simulink model "uz_ssi_interface"  (R2021a)
settings: Solver=FixedStepDiscrete  StartTime=0.0  StopTime=1200e-6  RelTol=1e-3
values from neighbouring files (symbols this model uses):
  f_ADC = 50e3    (= 50000)    [uz_ssi_interface_init.m]
  f_clock = 100e6    (= 100000000)    [uz_ssi_interface_init.m]
  ssi_encoder_bit_width = 17    [uz_ssi_interface_init.m]
  t_clock = 1/f_clock    (= 1e-08)    [uz_ssi_interface_init.m]
libraries: hdlsllib x21, simulink x10, simulink_extras x3, dspsigops x1
settings Model: DataTypeOverride=Off  Creator=micha  LastModifiedBy=micha
settings SolverCC: AlgebraicLoopSolver=TrustRegion
settings DataIOCC: LimitDataPoints=on  SaveOutput=off  SaveTime=off
settings OptimizationCC: BlockReduction=off  ConditionallyExecuteInputs=off  DefaultParameterBehavior=Inlined  LifeSpan=inf
settings DebuggingCC: AlgebraicLoopMsg=error  SingleTaskRateTransMsg=error  AllowSymbolicDim=off  StrictBusMsg=ErrorOnBusTreatedAsVector  SFUnexpectedBacktrackingDiag=warning  SFNoUnconditionalDefaultTransitionDiag=warning  SFExecutionAtInitializationDiag=none  SFMachineParentedDataDiag=warning  ArithmeticOperatorsInVariantConditions=warning
settings HardwareCC: ProdBitPerPointer=32  ProdBitPerSizeT=32  ProdBitPerPtrDiffT=32  ProdLargestAtomicFloat=None  ProdIntDivRoundTo=Undefined  ProdEndianess=Unspecified  ProdWordSize=32  ProdHWDeviceType=ASIC/FPGA->ASIC/FPGA  ProdEqTarget=off
settings SFSimCC: SimUseLocalCustomCode=off  CustomCodeUndefinedFunction=UseInterfaceOnly
settings RTWCC: RTWUseLocalCustomCode=off
settings CodeAppCC: StateflowObjectComments=on
settings GRTTargetCC: TargetLangStandard=C89/C90 (ANSI)
settings ConfigComp: CovScope=ReferencedModels  CovMetricSettings=dw  CovSaveCumulativeToWorkspaceVar=on  CovSaveSingleToWorkspaceVar=on  CovExternalEMLEnable=off  CovSFcnEnable=off

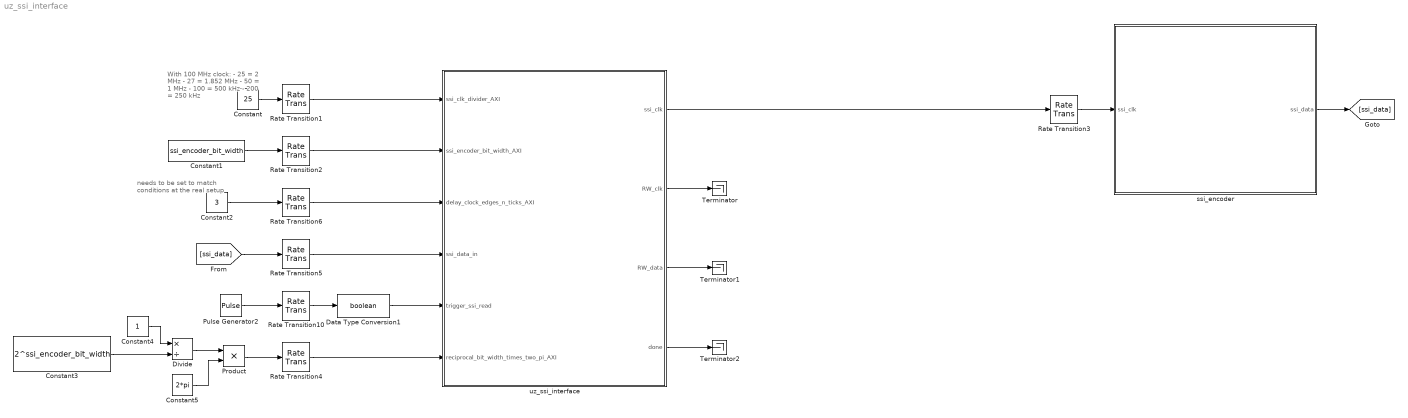
== system uz_ssi_interface ==
  note: With 100 MHz clock:
      |
      | -     25 = 2 MHz
      | -     27 = 1.852 MHz
      | -     50 = 1 MHz
      | -   100 = 500 kHz
      | -   200 = 250 kHz
  note: needs to be set to match conditions at
      |  the real setup
  Constant : Constant  Value=25  OutDataTypeStr=uint32  SampleTime=t_clock
  Constant1 : Constant  Value=ssi_encoder_bit_width  OutDataTypeStr=uint32  SampleTime=t_clock
  Constant2 : Constant  Value=3  OutDataTypeStr=uint32  SampleTime=t_clock
  Constant3 : Constant  Value=2^ssi_encoder_bit_width  OutDataTypeStr=single  SampleTime=t_clock
  Constant4 : Constant  OutDataTypeStr=single  SampleTime=t_clock
  Constant5 : Constant  Value=2*pi  OutDataTypeStr=single  SampleTime=t_clock
  Data Type Conversion1 : DataTypeConversion  OutDataTypeStr=boolean
  Divide : Product  Inputs=*/
  Product : Product
  Pulse Generator2 : DiscretePulseGenerator  Period=f_clock/f_ADC  PulseWidth=0.04*f_clock/f_ADC  SampleTime=t_clock
  Rate Transition{1..6,10} (7 alike) : RateTransition  OutPortSampleTime=t_clock
  Terminator : Terminator
  Terminator1 : Terminator
  Terminator2 : Terminator
  ssi_encoder : Subsystem
  uz_ssi_interface : Subsystem
  wires:
  Rate Transition10/1 -> Data Type Conversion1/1
  Pulse Generator2/1 -> Rate Transition10/1
  Data Type Conversion1/1 -> uz_ssi_interface/5(trigger_ssi_read)
  Constant/1 -> Rate Transition1/1
  Rate Transition1/1 -> uz_ssi_interface/1(ssi_clk_divider_AXI)
  Constant1/1 -> Rate Transition2/1
  Rate Transition2/1 -> uz_ssi_interface/2(ssi_encoder_bit_width_AXI)
  Rate Transition3/1 -> ssi_encoder/1(ssi_clk)
  ssi_encoder/1(ssi_data) -> [ssi_data]
  Rate Transition5/1 -> uz_ssi_interface/4(ssi_data_in)
  [ssi_data] -> Rate Transition5/1
  uz_ssi_interface/1(ssi_clk) -> Rate Transition3/1
  Rate Transition6/1 -> uz_ssi_interface/3(delay_clock_edges_n_ticks_AXI)
  Constant2/1 -> Rate Transition6/1
  uz_ssi_interface/3(RW_data) -> Terminator1/1
  uz_ssi_interface/4(done) -> Terminator2/1
  uz_ssi_interface/2(RW_clk) -> Terminator/1
  Rate Transition4/1 -> uz_ssi_interface/6(reciprocal_bit_width_times_two_pi_AXI)
  Product/1 -> Rate Transition4/1
  Divide/1 -> Product/1
  Constant4/1 -> Divide/1
  Constant3/1 -> Divide/2
  Constant5/1 -> Product/2

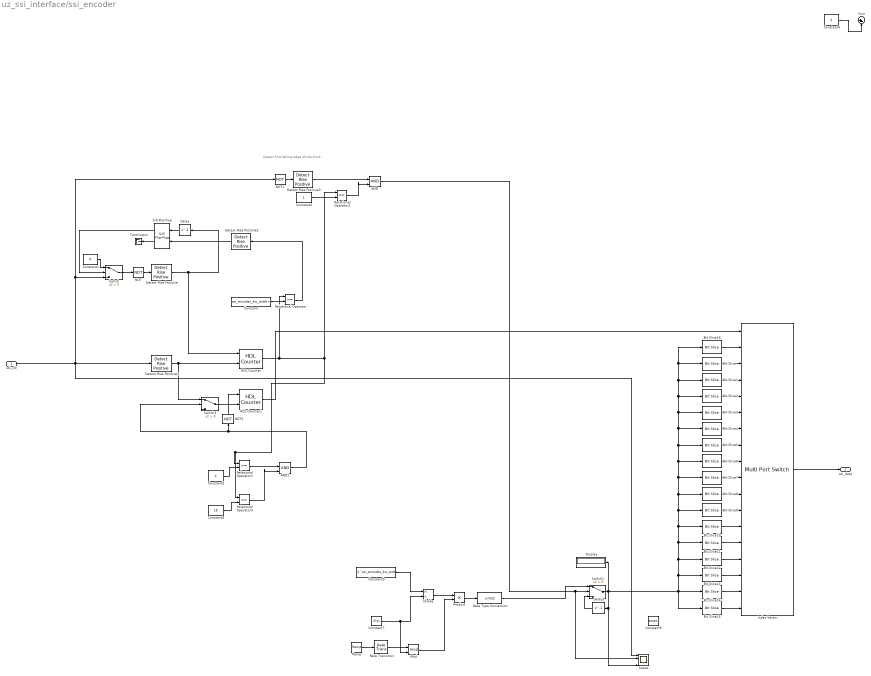
== system uz_ssi_interface/ssi_encoder ==
  note: Detect first falling edge of the clock
  ssi_clk : Inport
  AND : Logic  IconShape=distinctive  AllPortsSameDT=off  OutDataTypeStr=boolean
  AND1 : Logic  IconShape=distinctive  AllPortsSameDT=off  OutDataTypeStr=boolean
  Bit Slice : hdlsllib/Logic and Bit Operations/Bit Slice  lidx=15  ridx=15
      settings: SourceProductBaseCode=SL
  Bit Slice1 : hdlsllib/Logic and Bit Operations/Bit Slice  lidx=14  ridx=14
      settings: SourceProductBaseCode=SL
  Bit Slice10 : hdlsllib/Logic and Bit Operations/Bit Slice  lidx=5  ridx=5
      settings: SourceProductBaseCode=SL
  Bit Slice11 : hdlsllib/Logic and Bit Operations/Bit Slice  lidx=4  ridx=4
      settings: SourceProductBaseCode=SL
  Bit Slice12 : hdlsllib/Logic and Bit Operations/Bit Slice  lidx=3  ridx=3
      settings: SourceProductBaseCode=SL
  Bit Slice13 : hdlsllib/Logic and Bit Operations/Bit Slice  lidx=2  ridx=2
      settings: SourceProductBaseCode=SL
  Bit Slice14 : hdlsllib/Logic and Bit Operations/Bit Slice  lidx=1  ridx=1
      settings: SourceProductBaseCode=SL
  Bit Slice15 : hdlsllib/Logic and Bit Operations/Bit Slice  lidx=0  ridx=0
      settings: SourceProductBaseCode=SL
  Bit Slice16 : hdlsllib/Logic and Bit Operations/Bit Slice  lidx=16  ridx=16
      settings: SourceProductBaseCode=SL
  Bit Slice2 : hdlsllib/Logic and Bit Operations/Bit Slice  lidx=13  ridx=13
      settings: SourceProductBaseCode=SL
  Bit Slice3 : hdlsllib/Logic and Bit Operations/Bit Slice  lidx=12  ridx=12
      settings: SourceProductBaseCode=SL
  Bit Slice4 : hdlsllib/Logic and Bit Operations/Bit Slice  lidx=11  ridx=11
      settings: SourceProductBaseCode=SL
  Bit Slice5 : hdlsllib/Logic and Bit Operations/Bit Slice  lidx=10  ridx=10
      settings: SourceProductBaseCode=SL
  Bit Slice6 : hdlsllib/Logic and Bit Operations/Bit Slice  lidx=9  ridx=9
      settings: SourceProductBaseCode=SL
  Bit Slice7 : hdlsllib/Logic and Bit Operations/Bit Slice  lidx=8  ridx=8
      settings: SourceProductBaseCode=SL
  Bit Slice8 : hdlsllib/Logic and Bit Operations/Bit Slice  lidx=7  ridx=7
      settings: SourceProductBaseCode=SL
  Bit Slice9 : hdlsllib/Logic and Bit Operations/Bit Slice  lidx=6  ridx=6
      settings: SourceProductBaseCode=SL
  Constant : Constant  Value=ssi_encoder_bit_width+1  SampleTime=t_clock
  Constant1 : Constant  Value=0  SampleTime=t_clock
  Constant2 : Constant  SampleTime=t_clock
  Constant4 : Constant  Value=2  SampleTime=t_clock
  Constant5 : Constant  Value=2  SampleTime=t_clock
  Constant6 : Constant  Value=91329  OutDataTypeStr=uint32  SampleTime=t_clock
  Constant7 : Constant  Value=2*pi  SampleTime=t_clock
  Constant8 : Constant  Value=18  SampleTime=t_clock
  Constant9 : Constant  Value=2^ssi_encoder_bit_width  SampleTime=t_clock
  Data Type Conversion : DataTypeConversion  OutDataTypeStr=uint32
  Delay : Delay  DelayLength=1
  Delay2 : Delay  DelayLength=1  SampleTime=t_clock
  Detect Rise Positive{,1..3} (4 alike) : simulink/Logic and Bit Operations/Detect Rise Positive  vinit=0  OutDataTypeStr=boolean
  Display : Display
  Divide : Product  Inputs=*/
  HDL Counter : hdlsllib/Sources/HDL Counter  CountType=Count limited  CountInit=0  CountStep=1  CountMax=ssi_encoder_bit_width+1  CountFromType=Initial value  CountFrom=0  CountResetPort=on  CountLoadPort=off  CountEnbPort=on  CountDirPort=off  CountHitOutputPort=off  CountDataType=Unsigned  CountWordLen=8  CountFracLen=0  CountSampTime=t_clock
  HDL Counter1 : hdlsllib/Sources/HDL Counter  CountType=Count limited  CountInit=0  CountStep=1  CountMax=ssi_encoder_bit_width-1  CountFromType=Initial value  CountFrom=0  CountResetPort=on  CountLoadPort=off  CountEnbPort=on  CountDirPort=off  CountHitOutputPort=off  CountDataType=Unsigned  CountWordLen=8  CountFracLen=0  CountSampTime=t_clock
  Index Vector : MultiPortSwitch  DataPortOrder=Zero-based contiguous  Inputs=17  zeroidx=on
  Mod : Math  Operator=mod  SaturateOnIntegerOverflow=on
  NOT : Logic  Operator=NOT  IconShape=distinctive  AllPortsSameDT=off  OutDataTypeStr=boolean
  NOT1 : Logic  Operator=NOT  IconShape=distinctive  AllPortsSameDT=off  OutDataTypeStr=boolean
  NOT2 : Logic  Operator=NOT  IconShape=distinctive  AllPortsSameDT=off  OutDataTypeStr=boolean
  Product : Product
  Ramp : simulink/Sources/Ramp  slope=2*pi*1000  start=0  InitialOutput=0
  Rate Transition : RateTransition  OutPortSampleTime=t_clock
  Relational Operator : RelationalOperator  OutDataTypeStr=boolean  RndMeth=Simplest
  Relational Operator1 : RelationalOperator  OutDataTypeStr=boolean  RndMeth=Simplest
  Relational Operator2 : RelationalOperator  Operator===  OutDataTypeStr=boolean  RndMeth=Simplest
  Relational Operator3 : RelationalOperator  Operator=<=  OutDataTypeStr=boolean  RndMeth=Simplest
  S-R Flip-Flop : simulink_extras/Flip Flops/S-R Flip-Flop  initial_condition=0
  Scope : Scope  NumInputPorts=4
  Sum : Sum  Inputs=|+-
  Switch : Switch  Criteria=u2 > Threshold
  Switch1 : Switch  Criteria=u2 > Threshold
  Switch3 : Switch  Criteria=u2 > Threshold
  Terminator : Terminator
  ssi_data : Outport
  wires:
  NOT/1 -> Detect Rise Positive/1
  Constant/1 -> Relational Operator/2
  Switch/1 -> NOT/1
  S-R Flip-Flop/1 -> Switch/2
  Delay/1 -> S-R Flip-Flop/1
  Relational Operator/1 -> Detect Rise Positive2/1
  Detect Rise Positive2/1 -> S-R Flip-Flop/2
  Detect Rise Positive/1 -> HDL Counter/1, Delay/1
  Relational Operator2/1 -> AND/2
  Constant2/1 -> Relational Operator2/2
  NOT1/1 -> Detect Rise Positive3/1
  Detect Rise Positive3/1 -> AND/1
  Bit Slice16/1 -> Index Vector/2
  Bit Slice/1 -> Index Vector/3
  Bit Slice1/1 -> Index Vector/4
  Bit Slice2/1 -> Index Vector/5
  Bit Slice3/1 -> Index Vector/6
  Bit Slice4/1 -> Index Vector/7
  Bit Slice5/1 -> Index Vector/8
  Bit Slice6/1 -> Index Vector/9
  Bit Slice7/1 -> Index Vector/10
  Bit Slice8/1 -> Index Vector/11
  Bit Slice9/1 -> Index Vector/12
  Bit Slice10/1 -> Index Vector/13
  Bit Slice11/1 -> Index Vector/14
  Bit Slice12/1 -> Index Vector/15
  Bit Slice13/1 -> Index Vector/16
  Bit Slice14/1 -> Index Vector/17
  Bit Slice15/1 -> Index Vector/18
  Detect Rise Positive1/1 -> HDL Counter/2, Switch3/1
  HDL Counter/1 -> Relational Operator3/1, Relational Operator1/1, Relational Operator2/1, Relational Operator/1
  S-R Flip-Flop/2 -> Terminator/1
  Constant1/1 -> Switch/1
  ssi_clk/1 -> Scope/1, NOT1/1, Switch/3, Detect Rise Positive1/1
  Relational Operator1/1 -> AND1/1
  AND1/1 -> NOT2/1, Switch3/2
  Constant5/1 -> Relational Operator1/2
  Relational Operator3/1 -> AND1/2
  Constant8/1 -> Relational Operator3/2
  Constant4/1 -> Sum/2
  Switch3/1 -> HDL Counter1/2
  HDL Counter1/1 -> Index Vector/1
  NOT2/1 -> HDL Counter1/1
  Index Vector/1 -> ssi_data/1
  Ramp/1 -> Rate Transition/1
  Constant9/1 -> Divide/1
  Divide/1 -> Product/1
  Constant7/1 -> Mod/2, Divide/2
  Mod/1 -> Product/2
  Product/1 -> Data Type Conversion/1
  Rate Transition/1 -> Mod/1
  Delay2/1 -> Switch1/3
  Data Type Conversion/1 -> Switch1/1
  AND/1 -> Scope/2, Switch1/2
  Switch1/1 -> Bit Slice16/1, Bit Slice/1, Bit Slice1/1, Bit Slice2/1, Bit Slice3/1, Bit Slice4/1, Bit Slice5/1, Bit Slice6/1, Bit Slice7/1, Bit Slice8/1, Bit Slice9/1, Bit Slice10/1, Bit Slice11/1, Bit Slice12/1, Bit Slice13/1, Bit Slice15/1, Bit Slice14/1, Delay2/1, Scope/4, Display/1
  ? -> Scope/3

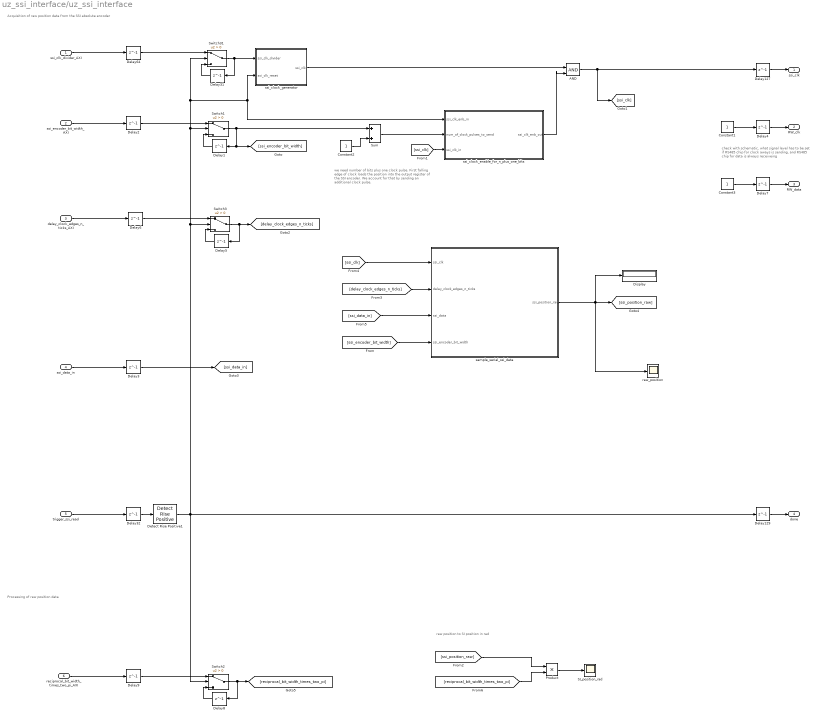
== system uz_ssi_interface/uz_ssi_interface ==
  note: raw position to SI position in rad
  note: Processing of raw position data
  note: check with schematic, what signal level has to be set if RS485 chip for clock aways is sending, and RS485 chip for data is always receiveing
  note: we need number of bits plus one clock pulse.
      | First falling edge of clock loads the position into the
      | output register of the SSI encoder. We account for that
      | by sending an additional clock pulse.
  note: Acquisition of raw position data from the SSI absolute encoder
  ssi_clk_divider_AXI : Inport  OutDataTypeStr=uint32
  ssi_encoder_bit_width_AXI : Inport  Port=2  OutDataTypeStr=uint32
  delay_clock_edges_n_ticks_AXI : Inport  Port=3  OutDataTypeStr=uint32
  ssi_data_in : Inport  Port=4
  trigger_ssi_read : Inport  Port=5  OutDataTypeStr=boolean
  reciprocal_bit_width_times_two_pi_AXI : Inport  Port=6  OutDataTypeStr=single
  AND : Logic  IconShape=distinctive  AllPortsSameDT=off  OutDataTypeStr=boolean
  Constant1 : Constant  OutDataTypeStr=boolean  SampleTime=t_clock
  Constant2 : Constant  OutDataTypeStr=uint32  SampleTime=t_clock
  Constant3 : Constant  OutDataTypeStr=boolean  SampleTime=t_clock
  Delay{1..9,31..32,64,127,129} (14 alike) : Delay  DelayLength=1
  Detect Rise Positive1 : simulink/Logic and Bit Operations/Detect Rise Positive  vinit=0  OutDataTypeStr=boolean
  Display : Display
  Product : Product
  SI_position_rad : Scope
  Sum : Sum  AccumDataTypeStr=uint32
  Switch{1..3,31} (4 alike) : Switch  Criteria=u2 > Threshold
  raw_position : Scope
  sample_serial_ssi_data : Subsystem
  ssi_clock_enable_for_n_plus_one_bits : Subsystem
  ssi_clock_generator : Subsystem
  ssi_clk : Outport
  RW_clk : Outport  Port=2
  RW_data : Outport  Port=3
  done : Outport  Port=4  OutDataTypeStr=boolean  LockScale=on
  wires:
  Delay129/1 -> done/1
  trigger_ssi_read/1 -> Delay32/1
  Delay32/1 -> Detect Rise Positive1/1
  Delay64/1 -> Switch31/1
  ssi_clk_divider_AXI/1 -> Delay64/1
  Delay31/1 -> Switch31/3
  Switch31/1 -> Delay31/1, ssi_clock_generator/1(ssi_clk_divider)
  ssi_clock_generator/1(ssi_clk) -> AND/1
  Switch1/1 -> Sum/1, [ssi_encoder_bit_width], Delay1/1
  Delay1/1 -> Switch1/3
  ssi_encoder_bit_width_AXI/1 -> Delay2/1
  Delay2/1 -> Switch1/1
  Constant2/1 -> Sum/2
  Sum/1 -> ssi_clock_enable_for_n_plus_one_bits/2(num_of_clock_pulses_to_send)
  ssi_clock_enable_for_n_plus_one_bits/1(ssi_clk_enb_out) -> AND/2
  AND/1 -> [ssi_clk], Delay127/1
  ssi_data_in/1 -> Delay3/1
  Delay127/1 -> ssi_clk/1
  [ssi_clk] -> ssi_clock_enable_for_n_plus_one_bits/3(ssi_clk_in)
  Delay5/1 -> Switch3/3
  Detect Rise Positive1/1 -> Switch2/2, Switch3/2, Switch31/2, ssi_clock_enable_for_n_plus_one_bits/1(ssi_clk_enb_in), ssi_clock_generator/2(ssi_clk_reset), Switch1/2, Delay129/1
  Delay6/1 -> Switch3/1
  delay_clock_edges_n_ticks_AXI/1 -> Delay6/1
  Switch3/1 -> Delay5/1, [delay_clock_edges_n_ticks]
  Delay3/1 -> [ssi_data_in]
  [ssi_clk] -> sample_serial_ssi_data/1(ssi_clk)
  [delay_clock_edges_n_ticks] -> sample_serial_ssi_data/2(delay_clock_edges_n_ticks)
  [ssi_data_in] -> sample_serial_ssi_data/3(ssi_data)
  sample_serial_ssi_data/1(ssi_position_raw) -> raw_position/1, [ssi_position_raw], Display/1
  [ssi_encoder_bit_width] -> sample_serial_ssi_data/4(ssi_encoder_bit_width)
  Delay4/1 -> RW_clk/1
  Delay7/1 -> RW_data/1
  Constant1/1 -> Delay4/1
  Constant3/1 -> Delay7/1
  [ssi_position_raw] -> Product/1
  [reciprocal_bit_width_times_two_pi] -> Product/2
  Product/1 -> SI_position_rad/1
  reciprocal_bit_width_times_two_pi_AXI/1 -> Delay9/1
  Switch2/1 -> Delay8/1, [reciprocal_bit_width_times_two_pi]
  Delay9/1 -> Switch2/1
  Delay8/1 -> Switch2/3

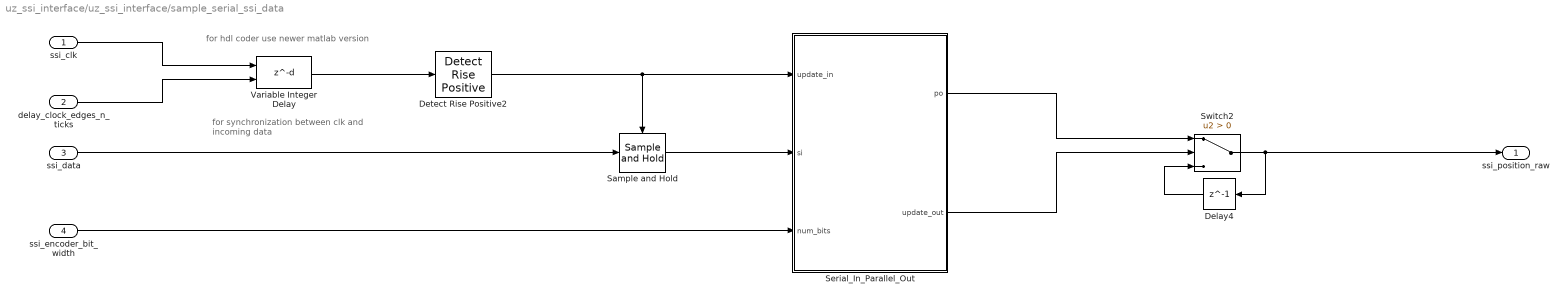
== system uz_ssi_interface/uz_ssi_interface/sample_serial_ssi_data ==
  note: for hdl coder use newer matlab version
  note: for synchronization between clk and
      | incoming data
  ssi_clk : Inport
  delay_clock_edges_n_ticks : Inport  Port=2
  ssi_data : Inport  Port=3
  ssi_encoder_bit_width : Inport  Port=4
  Delay4 : Delay  DelayLength=1
  Detect Rise Positive2 : simulink/Logic and Bit Operations/Detect Rise Positive  vinit=0  OutDataTypeStr=boolean
  Sample and Hold : dspsigops/Sample and Hold  trig=Rising edge  initCond=0  latchinput=off
  Serial_In_Parallel_Out : MATLAB Function  TreatAsAtomicUnit=on
  Switch2 : Switch  Criteria=u2 > Threshold
  Variable Integer Delay : Delay  DelayLengthSource=Input port  SampleTime=t_clock
      settings: InputPortMap=u0,p1
  ssi_position_raw : Outport
  wires:
  Variable Integer Delay/1 -> Detect Rise Positive2/1
  delay_clock_edges_n_ticks/1 -> Variable Integer Delay/2
  Delay4/1 -> Switch2/3
  Sample and Hold/1 -> Serial_In_Parallel_Out/2(si)
  Serial_In_Parallel_Out/2(update_out) -> Switch2/2
  ssi_encoder_bit_width/1 -> Serial_In_Parallel_Out/3(num_bits)
  Serial_In_Parallel_Out/1(po) -> Switch2/1
  Detect Rise Positive2/1 -> Sample and Hold/Trigger, Serial_In_Parallel_Out/1(update_in)
  ssi_data/1 -> Sample and Hold/1
  Switch2/1 -> ssi_position_raw/1, Delay4/1
  ssi_clk/1 -> Variable Integer Delay/1

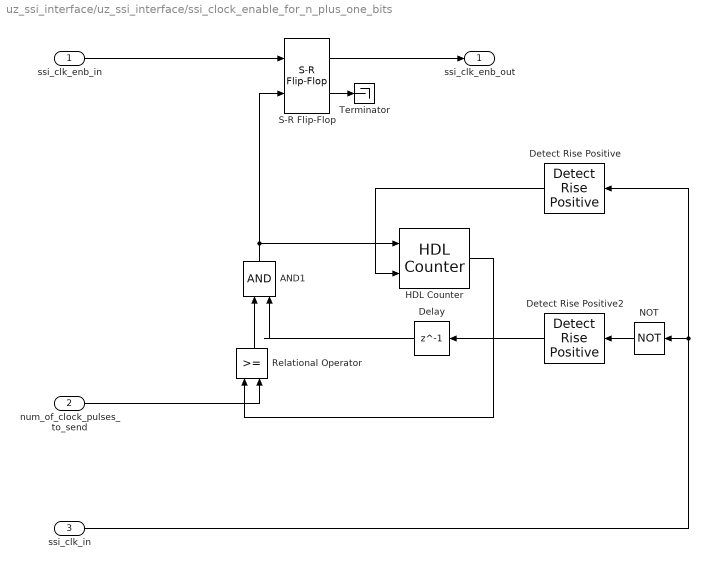
== system uz_ssi_interface/uz_ssi_interface/ssi_clock_enable_for_n_plus_one_bits ==
  ssi_clk_enb_in : Inport
  num_of_clock_pulses_to_send : Inport  Port=2
  ssi_clk_in : Inport  Port=3
  AND1 : Logic  IconShape=distinctive  AllPortsSameDT=off  OutDataTypeStr=boolean
  Delay : Delay  DelayLength=1
  Detect Rise Positive : simulink/Logic and Bit Operations/Detect Rise Positive  vinit=0  OutDataTypeStr=boolean
  Detect Rise Positive2 : simulink/Logic and Bit Operations/Detect Rise Positive  vinit=0  OutDataTypeStr=boolean
  HDL Counter : hdlsllib/Sources/HDL Counter  CountType=Free running  CountInit=0  CountStep=1  CountMax=25  CountFromType=Initial value  CountFrom=0  CountResetPort=on  CountLoadPort=off  CountEnbPort=on  CountDirPort=off  CountHitOutputPort=off  CountDataType=Unsigned  CountWordLen=8  CountFracLen=0  CountSampTime=1
  NOT : Logic  Operator=NOT  IconShape=distinctive  AllPortsSameDT=off  OutDataTypeStr=boolean
  Relational Operator : RelationalOperator  OutDataTypeStr=boolean  RndMeth=Simplest
  S-R Flip-Flop : simulink_extras/Flip Flops/S-R Flip-Flop  initial_condition=0
  Terminator : Terminator
  ssi_clk_enb_out : Outport
  wires:
  HDL Counter/1 -> Relational Operator/1
  num_of_clock_pulses_to_send/1 -> Relational Operator/2
  Detect Rise Positive2/1 -> Delay/1
  S-R Flip-Flop/2 -> Terminator/1
  Relational Operator/1 -> AND1/1
  Detect Rise Positive/1 -> HDL Counter/2
  AND1/1 -> HDL Counter/1, S-R Flip-Flop/2
  ssi_clk_in/1 -> Detect Rise Positive/1, NOT/1
  NOT/1 -> Detect Rise Positive2/1
  ssi_clk_enb_in/1 -> S-R Flip-Flop/1
  S-R Flip-Flop/1 -> ssi_clk_enb_out/1
  Delay/1 -> AND1/2

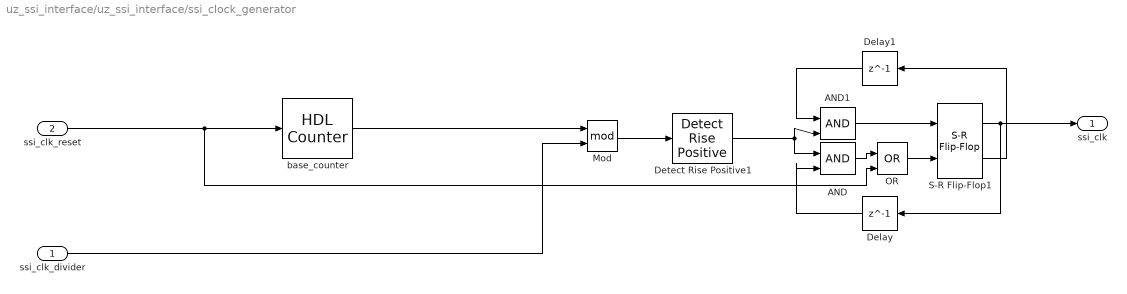
== system uz_ssi_interface/uz_ssi_interface/ssi_clock_generator ==
  ssi_clk_divider : Inport
  ssi_clk_reset : Inport  Port=2
  AND : Logic  IconShape=distinctive  AllPortsSameDT=off  OutDataTypeStr=boolean
  AND1 : Logic  IconShape=distinctive  AllPortsSameDT=off  OutDataTypeStr=boolean
  Delay : Delay  DelayLength=1
  Delay1 : Delay  DelayLength=1
  Detect Rise Positive1 : simulink/Logic and Bit Operations/Detect Rise Positive  vinit=0  OutDataTypeStr=boolean
  Mod : Math  Operator=mod  SaturateOnIntegerOverflow=on
  OR : Logic  Operator=OR  IconShape=distinctive  AllPortsSameDT=off  OutDataTypeStr=boolean
  S-R Flip-Flop1 : simulink_extras/Flip Flops/S-R Flip-Flop  initial_condition=0
  base_counter : hdlsllib/Sources/HDL Counter  CountType=Free running  CountInit=0  CountStep=1  CountMax=199  CountFromType=Initial value  CountFrom=0  CountResetPort=on  CountLoadPort=off  CountEnbPort=off  CountDirPort=off  CountHitOutputPort=off  CountDataType=Unsigned  CountWordLen=16  CountFracLen=0  CountSampTime=1
  ssi_clk : Outport
  wires:
  base_counter/1 -> Mod/1
  ssi_clk_divider/1 -> Mod/2
  Mod/1 -> Detect Rise Positive1/1
  ssi_clk_reset/1 -> OR/2, base_counter/1
  Detect Rise Positive1/1 -> AND1/2, AND/1
  S-R Flip-Flop1/1 -> ssi_clk/1, Delay/1
  AND1/1 -> S-R Flip-Flop1/1
  S-R Flip-Flop1/2 -> Delay1/1
  Delay/1 -> AND/2
  Delay1/1 -> AND1/1
  OR/1 -> S-R Flip-Flop1/2
  AND/1 -> OR/1

== matlab function uz_ssi_interface/sample_serial_ssi_data/Serial_In_Parallel_Out ==
  data: po output; update_in input; update_out output; si input; num_bits input
function [po, update_out] = SIPO(update_in, si, num_bits)
%#codegen

max_bits = 32;  % Maximum number of bits (fixed to 32 bits for all variables)

persistent parallel_out ...
    regout ...
    count_bits % Count the bits being output

if isempty(parallel_out)
    % Always initialize as 32-bit fixed-point numbers
    parallel_out = fi(0, 0, max_bits, 0);  % 32-bit parallel output
    regout = fi(0, 0, max_bits, 0);         % 32-bit register output
    count_bits = fi(0, 0, ceil(log2(max_bits)) + 1, 0);  % 32-bit counter
end

% Set the output parallel register as a fixed-point object (32 bits)
po = fi(0, 0, max_bits, 0);  % Parallel output of width 32 bits
po(:) = regout;  % Register output
update_out = fi(0, 0, 1, 0);  % Binary update output (1-bit)

if update_in == 1
    % The actual shift register here.
    % Join the old with the new
    % by dropping the MSB and keeping the bits below this to the LSB.
    % and appending the si input to the LSB.
    
    % We are concatenating and shifting
    parallel_out(:) = bitconcat(...
        bitsliceget(parallel_out, max_bits - 1, 1), ...  % Get the MSB to LSB bits (constant indices)
        fi(si, 0, 1, 0));  % Append the new input `si`
    
    % Mask the result to the number of bits specified by num_bits
    % Create a mask for the desired number of bits (this is a constant)
    mask = fi(2^num_bits - 1, 0, max_bits, 0);  % Create a mask with 'num_bits' set to 1
    
    % Apply the mask to parallel_out to keep only the lower 'num_bits'
    parallel_out = bitand(parallel_out, mask);  % Apply bitwise AND
    
    if count_bits >= num_bits
        regout(:) = parallel_out;  % Update the register with the parallel output
        update_out = fi(1, 0, 1, 0);  % There has been an output
        count_bits(:) = 0;  % Reset the counter
    else
        count_bits(:) = count_bits + 1;  % Increment the counter
    end
end
